simulink model "VN1610_minimal_example"  (R2021b)
settings: Solver=FixedStepDiscrete  StartTime=0.0  StopTime=Inf  RelTol=1e-3
undefined symbols (not defined in the file): canChannel
libraries: canlib x3, canmsglib x2
settings Model: Creator=mfussi  LastModifiedBy=mfussi

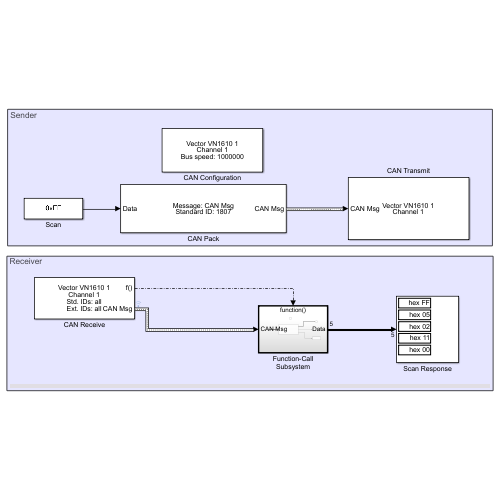
[thumbnail: Simulink's stored preview of the top-level diagram]
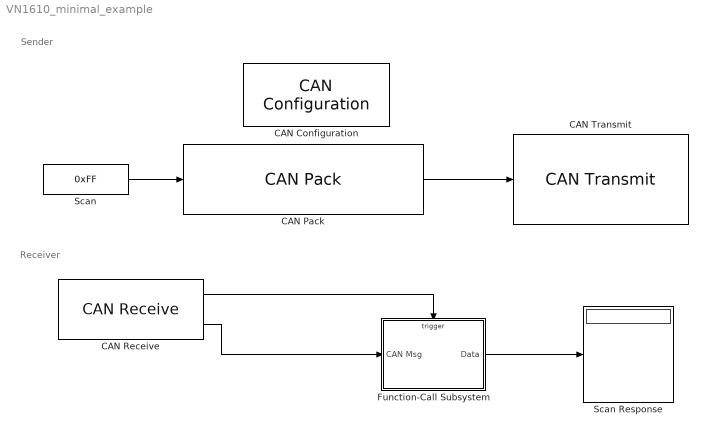
== system VN1610_minimal_example ==
  note: Sender
  note: Receiver
  CAN Configuration : canlib/CAN Configuration  BlockHandle=2.0001  Device=Vector VN1610 1 (Channel 1)  DeviceMenu=Vector VN1610 1 (Channel 1)  ObjConstructor=canChannel('Vector', 'VN1610 1', 1)  BusSpeed=1000000  EnableBitParameters=off  SJW=1  TSEG1=4  TSEG2=3  NSamples=1  AckMode=Normal
      settings: SourceProductBaseCode=VN
  CAN Pack : canmsglib/CAN Pack  MsgList=(none)  MsgName=CAN Msg  MsgIDType=Standard (11-bit identifier)  MsgIdentifier=1807  MsgLength=1  Remote=off  ApplyMinMax=off  BusOutput=on  SignalInfo={}
      settings: SourceProductBaseCode=ME,XP,VN  DataFormat=raw data
  CAN Receive : canlib/CAN Receive  BlockHandle=4.0001  Device=Vector VN1610 1 (Channel 1)  DeviceMenu=Vector VN1610 1 (Channel 1)  ObjConstructor=canChannel('Vector', 'VN1610 1', 1)  EnableStandardIDsFilter=off  StdIDsCombo=Allow all  StandardIDs=0  EnableExtendedIDsFilter=off  ExtIDsCombo=Allow all  ExtendedIDs=0  SampleTime=0.01  MsgsPerTimestep=all  InternalFilterUpdateStatus=on  BusOutput=on
      settings: SourceProductBaseCode=VN
  CAN Transmit : canlib/CAN Transmit  BlockHandle=5.0001  Device=Vector VN1610 1 (Channel 1)  DeviceMenu=Vector VN1610 1 (Channel 1)  ObjConstructor=canChannel('Vector', 'VN1610 1', 1)  EnableEventTransmit=off  EnablePeriodicTransmit=off  MessagePeriod=1.000
      settings: SourceProductBaseCode=VN
  Function-Call Subsystem : Subsystem  TreatAsAtomicUnit=on
  Scan : Constant  Value=0xFF
  Scan Response : Display
      settings: Format=hex (Stored Integer)
  wires:
  CAN Pack/1 -> CAN Transmit/1
  CAN Receive/1 -> Function-Call Subsystem/Trigger
  CAN Receive/2 -> Function-Call Subsystem/1(CAN Msg)
  Scan/1 -> CAN Pack/1
  Function-Call Subsystem/1(Data) -> Scan Response/1

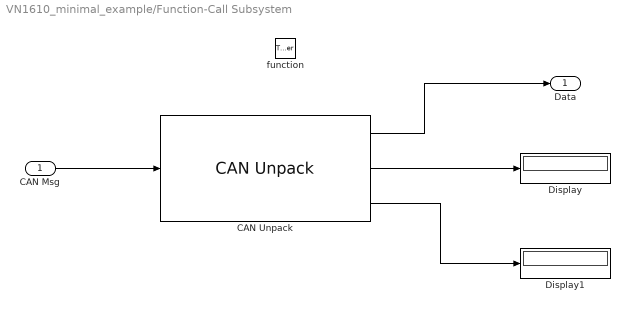
== system VN1610_minimal_example/Function-Call Subsystem ==
  CAN Msg : Inport
  function : TriggerPort  TriggerType=function-call  VariantControl=(inherit)
  CAN Unpack : canmsglib/CAN Unpack  MsgList=(none)  MsgName=CAN Msg  MsgIDType=Standard (11-bit identifier)  MsgIdentifier=1824  MsgLength=5  SignalInfo={}  IDPort=off  TimestampPort=on  ErrorPort=off  RemotePort=off  LengthPort=on  StatusPort=off  ApplyMinMax=off
      settings: SourceProductBaseCode=ME,XP,VN  DataFormat=raw data
  Display : Display
  Display1 : Display
  Data : Outport
  wires:
  CAN Msg/1 -> CAN Unpack/1
  CAN Unpack/1 -> Data/1
  CAN Unpack/2 -> Display/1
  CAN Unpack/3 -> Display1/1
